simulink model "TL"  (R2013a)
settings: Solver=ode45  StartTime=0.0  StopTime=200  RelTol=1e-3
settings Model: Creator=Ahmed  LastModifiedBy=Ahmed

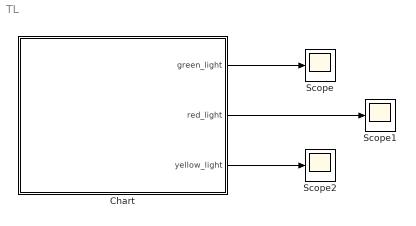
== system TL ==
  Chart : Stateflow chart  TreatAsAtomicUnit=on
  Scope : Scope
  Scope1 : Scope
  Scope2 : Scope
      settings: SaveName=ScopeData2
  wires:
  Chart/1(green_light) -> Scope/1
  Chart/2(red_light) -> Scope1/1
  Chart/3(yellow_light) -> Scope2/1

== stateflow chart TL/Chart ==
  state RED
    entry:
    red_light=1;
    yellow_light=0;
    green_light=0;
  state GREEN
    entry:
    red_light=0;
    yellow_light=0;
    green_light=1;
  state YELLOW
    entry:
    red_light=0;
    yellow_light=1;
    green_light=0;
  (default) -> RED
  RED -> GREEN : after(50,sec)
  YELLOW -> RED : after(5,sec)
  GREEN -> YELLOW : after(40,sec)
  data: green_light output double; red_light output double; yellow_light output double
